simulink model "frbd_64ch_600mhz"  (R2013b)
settings: Solver=FixedStepDiscrete  SolverMode=SingleTasking  StartTime=0.0  StopTime=10.0  RelTol=1e-3
undefined symbols (not defined in the file): pfb_coeff_gen_calc
libraries: xbsIndex_r4 x14825, casper_library_delays x97, casper_library_misc x66, dspsigops x16, xps_library x5, casper_library_pfbs x2
(part 6 of 149)

== system frbd_64ch_600mhz/ACC6 ==
  addr : Inport
  data_in : Inport  Port=2
  we : Inport  Port=3
  calc_add : Subsystem  mask{data_width=32, addr_width=10, sample_rate=sample_rate}
      mask prompts: data_width "data width"; addr_width "address width"; sample_rate "sample rate"
  convert_addr : xbsIndex_r4/Convert  gui_display_data_type=Fixed-point  arith_type=Unsigned  n_bits=addr_width  bin_pt=0  float_type=Single  exp_bits=8  fraction_bits=24  quantization=Truncate  overflow=Wrap  en=off  latency=0  dbl_ovrd=off  pipeline=off  block_type=convert
      settings: xl_area=[0, 0, 0, 0, 0, 0, 0]
  convert_din1 : xbsIndex_r4/Convert  gui_display_data_type=Fixed-point  arith_type=Unsigned  n_bits=32  bin_pt=0  float_type=Single  exp_bits=8  fraction_bits=24  quantization=Truncate  overflow=Wrap  en=off  latency=0  dbl_ovrd=off  pipeline=off  block_type=convert
      settings: xl_area=[0, 0, 0, 0, 0, 0, 0]
  convert_we : xbsIndex_r4/Convert  gui_display_data_type=Fixed-point  arith_type=Unsigned  n_bits=1  bin_pt=0  float_type=Single  exp_bits=8  fraction_bits=24  quantization=Truncate  overflow=Wrap  en=off  latency=0  dbl_ovrd=off  pipeline=off  block_type=convert
      settings: xl_area=[0, 0, 0, 0, 0, 0, 0]
  frbd_64ch_600mhz_ACC6_addr : xbsIndex_r4/Gateway Out  inherit_from_input=off  hdl_port=on  timing_constraint=None  locs_specified=off  LOCs={'A5','B9','A9','C1','A3','G6','E9','A6','A7','A8','B8','B1','B3','D9','B5','B4','B6','C2'}  UseAsDAC=off  DACChannel='1'  block_type=gatewayout
      settings: infoedit="Gateway out block.  Converts Xilinx fixed point inputs into ouputs of type Simulink integer, double, or fixed point.<P><P>Hardware notes:  In hardware these blocks become top level output ports or are discarded, depending on how they are configured."  xl_area=[0, 0, 0, 0, 0, 0, 0]  sginterface={'Nallatech'=>{'xdspkit'=>{'non_memory_mapped_port'=>'uprev_Shared_BRAM_addr'}},'Xilinx'=>{'jtaghwcosim'=>{'non_memory_mapped_port'=>'uprev_Shared_BRAM_addr'},'xdspkit'=>{'non_memory_mapped_port'=>'uprev_Shared_BRAM_addr'}}}
  frbd_64ch_600mhz_ACC6_data_in : xbsIndex_r4/Gateway Out  inherit_from_input=off  hdl_port=on  timing_constraint=None  locs_specified=off  LOCs={'B21','B22','A22','B23','B19','C19','A20','A21','A23','B24','A24','A25','E18','D18','C18','B18'}  UseAsDAC=off  DACChannel='1'  block_type=gatewayout
      settings: infoedit="Gateway out block.  Converts Xilinx fixed point inputs into ouputs of type Simulink integer, double, or fixed point.<P><P>Hardware notes:  In hardware these blocks become top level output ports or are discarded, depending on how they are configured."  xl_area=[0, 0, 0, 0, 0, 0, 0]  sginterface={'Nallatech'=>{'xdspkit'=>{'non_memory_mapped_port'=>'uprev_Shared_BRAM_data_in'}},'Xilinx'=>{'jtaghwcosim'=>{'non_memory_mapped_port'=>'uprev_Shared_BRAM_data_in'},'xdspkit'=>{'non_memory_mapped_port'=>'uprev_Shared_BRAM_data_in'}}}
  frbd_64ch_600mhz_ACC6_data_out : xbsIndex_r4/Gateway In  gui_display_data_type=Fixed-point  arith_type=Unsigned  n_bits=32  bin_pt=0  preci_type=Single  exp_width=8  frac_width=24  quantization=Truncate  overflow=Wrap  period=sample_rate  dbl_ovrd=off  timing_constraint=None  locs_specified=off  LOCs={}  UseAsADC=off  ADCChannel='1'  inherit_from_input=off  hdl_port=on  block_type=gatewayin
      settings: xl_area=[0, 0, 0, 0, 0, 0, 0]
  frbd_64ch_600mhz_ACC6_we : xbsIndex_r4/Gateway Out  inherit_from_input=off  hdl_port=on  timing_constraint=None  locs_specified=off  LOCs={'A14'}  UseAsDAC=off  DACChannel='1'  block_type=gatewayout
      settings: infoedit="Gateway out block.  Converts Xilinx fixed point inputs into ouputs of type Simulink integer, double, or fixed point.<P><P>Hardware notes:  In hardware these blocks become top level output ports or are discarded, depending on how they are configured."  xl_area=[0, 0, 0, 0, 0, 0, 0]
  mem : Subsystem
  munge_in : Subsystem  AncestorBlock=casper_library_flow_control/munge  mask(munge){divisions=1, div_size=32, order=[0], arith_type_out=Unsigned, bin_pt_out=0}
      mask prompts: divisions "Number of divisions"; div_size "Division size (bits)"; order "Division packing order"; arith_type_out "Output arithmetic type"; bin_pt_out "Output binary point"
      mask help: Splits an input bus into the specified number of divisions and then recombines them in the order specified (most significant division = 0,least = number divisions-1)
      mask init:
      | munge_init(gcb, ...
      |     'divisions', divisions, ...
      |     'div_size', div_size, ...
      |     'order', order, ...
      |     'arith_type_out', arith_type_out, ...
      |     'bin_pt_out', bin_pt_out);
      settings: AttributesFormatString=|
      | split:32
      | join:0
      | Unsigned [32,0]
      mask TypeOptions arith_type_out: Unsigned | Signed  (2's comp) | Floating-point
  munge_out : Subsystem  AncestorBlock=casper_library_flow_control/munge  mask(munge){divisions=1, div_size=32, order=[0], arith_type_out=Unsigned, bin_pt_out=0}
      mask prompts: divisions "Number of divisions"; div_size "Division size (bits)"; order "Division packing order"; arith_type_out "Output arithmetic type"; bin_pt_out "Output binary point"
      mask help: Splits an input bus into the specified number of divisions and then recombines them in the order specified (most significant division = 0,least = number divisions-1)
      mask init:
      | munge_init(gcb, ...
      |     'divisions', divisions, ...
      |     'div_size', div_size, ...
      |     'order', order, ...
      |     'arith_type_out', arith_type_out, ...
      |     'bin_pt_out', bin_pt_out);
      settings: AttributesFormatString=|
      | split:32
      | join:0
      | Unsigned [32,0]
      mask TypeOptions arith_type_out: Unsigned | Signed  (2's comp) | Floating-point
  data_out : Outport
  wires:
  munge_in/1(dout) -> convert_din1/1
  munge_out/1(dout) -> data_out/1
  we/1 -> convert_we/1
  addr/1 -> calc_add/1(in)
  mem/1(Out1) -> frbd_64ch_600mhz_ACC6_data_out/1
  frbd_64ch_600mhz_ACC6_data_out/1 -> munge_out/1(din)
  convert_we/1 -> frbd_64ch_600mhz_ACC6_we/1
  frbd_64ch_600mhz_ACC6_addr/1 -> mem/1(In1)
  frbd_64ch_600mhz_ACC6_data_in/1 -> mem/2(In2)
  frbd_64ch_600mhz_ACC6_we/1 -> mem/3(In3)
  calc_add/1(out) -> convert_addr/1
  data_in/1 -> munge_in/1(din)
  convert_din1/1 -> frbd_64ch_600mhz_ACC6_data_in/1
  convert_addr/1 -> frbd_64ch_600mhz_ACC6_addr/1

== system frbd_64ch_600mhz/ACC7 ==
  addr : Inport
  data_in : Inport  Port=2
  we : Inport  Port=3
  calc_add : Subsystem  mask{data_width=32, addr_width=10, sample_rate=sample_rate}
      mask prompts: data_width "data width"; addr_width "address width"; sample_rate "sample rate"
  convert_addr : xbsIndex_r4/Convert  gui_display_data_type=Fixed-point  arith_type=Unsigned  n_bits=addr_width  bin_pt=0  float_type=Single  exp_bits=8  fraction_bits=24  quantization=Truncate  overflow=Wrap  en=off  latency=0  dbl_ovrd=off  pipeline=off  block_type=convert
      settings: xl_area=[0, 0, 0, 0, 0, 0, 0]
  convert_din1 : xbsIndex_r4/Convert  gui_display_data_type=Fixed-point  arith_type=Unsigned  n_bits=32  bin_pt=0  float_type=Single  exp_bits=8  fraction_bits=24  quantization=Truncate  overflow=Wrap  en=off  latency=0  dbl_ovrd=off  pipeline=off  block_type=convert
      settings: xl_area=[0, 0, 0, 0, 0, 0, 0]
  convert_we : xbsIndex_r4/Convert  gui_display_data_type=Fixed-point  arith_type=Unsigned  n_bits=1  bin_pt=0  float_type=Single  exp_bits=8  fraction_bits=24  quantization=Truncate  overflow=Wrap  en=off  latency=0  dbl_ovrd=off  pipeline=off  block_type=convert
      settings: xl_area=[0, 0, 0, 0, 0, 0, 0]
  frbd_64ch_600mhz_ACC7_addr : xbsIndex_r4/Gateway Out  inherit_from_input=off  hdl_port=on  timing_constraint=None  locs_specified=off  LOCs={'A5','B9','A9','C1','A3','G6','E9','A6','A7','A8','B8','B1','B3','D9','B5','B4','B6','C2'}  UseAsDAC=off  DACChannel='1'  block_type=gatewayout
      settings: infoedit="Gateway out block.  Converts Xilinx fixed point inputs into ouputs of type Simulink integer, double, or fixed point.<P><P>Hardware notes:  In hardware these blocks become top level output ports or are discarded, depending on how they are configured."  xl_area=[0, 0, 0, 0, 0, 0, 0]  sginterface={'Nallatech'=>{'xdspkit'=>{'non_memory_mapped_port'=>'uprev_Shared_BRAM_addr'}},'Xilinx'=>{'jtaghwcosim'=>{'non_memory_mapped_port'=>'uprev_Shared_BRAM_addr'},'xdspkit'=>{'non_memory_mapped_port'=>'uprev_Shared_BRAM_addr'}}}
  frbd_64ch_600mhz_ACC7_data_in : xbsIndex_r4/Gateway Out  inherit_from_input=off  hdl_port=on  timing_constraint=None  locs_specified=off  LOCs={'B21','B22','A22','B23','B19','C19','A20','A21','A23','B24','A24','A25','E18','D18','C18','B18'}  UseAsDAC=off  DACChannel='1'  block_type=gatewayout
      settings: infoedit="Gateway out block.  Converts Xilinx fixed point inputs into ouputs of type Simulink integer, double, or fixed point.<P><P>Hardware notes:  In hardware these blocks become top level output ports or are discarded, depending on how they are configured."  xl_area=[0, 0, 0, 0, 0, 0, 0]  sginterface={'Nallatech'=>{'xdspkit'=>{'non_memory_mapped_port'=>'uprev_Shared_BRAM_data_in'}},'Xilinx'=>{'jtaghwcosim'=>{'non_memory_mapped_port'=>'uprev_Shared_BRAM_data_in'},'xdspkit'=>{'non_memory_mapped_port'=>'uprev_Shared_BRAM_data_in'}}}
  frbd_64ch_600mhz_ACC7_data_out : xbsIndex_r4/Gateway In  gui_display_data_type=Fixed-point  arith_type=Unsigned  n_bits=32  bin_pt=0  preci_type=Single  exp_width=8  frac_width=24  quantization=Truncate  overflow=Wrap  period=sample_rate  dbl_ovrd=off  timing_constraint=None  locs_specified=off  LOCs={}  UseAsADC=off  ADCChannel='1'  inherit_from_input=off  hdl_port=on  block_type=gatewayin
      settings: xl_area=[0, 0, 0, 0, 0, 0, 0]
  frbd_64ch_600mhz_ACC7_we : xbsIndex_r4/Gateway Out  inherit_from_input=off  hdl_port=on  timing_constraint=None  locs_specified=off  LOCs={'A14'}  UseAsDAC=off  DACChannel='1'  block_type=gatewayout
      settings: infoedit="Gateway out block.  Converts Xilinx fixed point inputs into ouputs of type Simulink integer, double, or fixed point.<P><P>Hardware notes:  In hardware these blocks become top level output ports or are discarded, depending on how they are configured."  xl_area=[0, 0, 0, 0, 0, 0, 0]
  mem : Subsystem
  munge_in : Subsystem  AncestorBlock=casper_library_flow_control/munge  mask(munge){divisions=1, div_size=32, order=[0], arith_type_out=Unsigned, bin_pt_out=0}
      mask prompts: divisions "Number of divisions"; div_size "Division size (bits)"; order "Division packing order"; arith_type_out "Output arithmetic type"; bin_pt_out "Output binary point"
      mask help: Splits an input bus into the specified number of divisions and then recombines them in the order specified (most significant division = 0,least = number divisions-1)
      mask init:
      | munge_init(gcb, ...
      |     'divisions', divisions, ...
      |     'div_size', div_size, ...
      |     'order', order, ...
      |     'arith_type_out', arith_type_out, ...
      |     'bin_pt_out', bin_pt_out);
      settings: AttributesFormatString=|
      | split:32
      | join:0
      | Unsigned [32,0]
      mask TypeOptions arith_type_out: Unsigned | Signed  (2's comp) | Floating-point
  munge_out : Subsystem  AncestorBlock=casper_library_flow_control/munge  mask(munge){divisions=1, div_size=32, order=[0], arith_type_out=Unsigned, bin_pt_out=0}
      mask prompts: divisions "Number of divisions"; div_size "Division size (bits)"; order "Division packing order"; arith_type_out "Output arithmetic type"; bin_pt_out "Output binary point"
      mask help: Splits an input bus into the specified number of divisions and then recombines them in the order specified (most significant division = 0,least = number divisions-1)
      mask init:
      | munge_init(gcb, ...
      |     'divisions', divisions, ...
      |     'div_size', div_size, ...
      |     'order', order, ...
      |     'arith_type_out', arith_type_out, ...
      |     'bin_pt_out', bin_pt_out);
      settings: AttributesFormatString=|
      | split:32
      | join:0
      | Unsigned [32,0]
      mask TypeOptions arith_type_out: Unsigned | Signed  (2's comp) | Floating-point
  data_out : Outport
  wires:
  munge_in/1(dout) -> convert_din1/1
  munge_out/1(dout) -> data_out/1
  we/1 -> convert_we/1
  addr/1 -> calc_add/1(in)
  mem/1(Out1) -> frbd_64ch_600mhz_ACC7_data_out/1
  frbd_64ch_600mhz_ACC7_data_out/1 -> munge_out/1(din)
  convert_we/1 -> frbd_64ch_600mhz_ACC7_we/1
  frbd_64ch_600mhz_ACC7_addr/1 -> mem/1(In1)
  frbd_64ch_600mhz_ACC7_data_in/1 -> mem/2(In2)
  frbd_64ch_600mhz_ACC7_we/1 -> mem/3(In3)
  calc_add/1(out) -> convert_addr/1
  data_in/1 -> munge_in/1(din)
  convert_din1/1 -> frbd_64ch_600mhz_ACC7_data_in/1
  convert_addr/1 -> frbd_64ch_600mhz_ACC7_addr/1

== system frbd_64ch_600mhz/ACC8 ==
  addr : Inport
  data_in : Inport  Port=2
  we : Inport  Port=3
  calc_add : Subsystem  mask{data_width=32, addr_width=10, sample_rate=sample_rate}
      mask prompts: data_width "data width"; addr_width "address width"; sample_rate "sample rate"
  convert_addr : xbsIndex_r4/Convert  gui_display_data_type=Fixed-point  arith_type=Unsigned  n_bits=addr_width  bin_pt=0  float_type=Single  exp_bits=8  fraction_bits=24  quantization=Truncate  overflow=Wrap  en=off  latency=0  dbl_ovrd=off  pipeline=off  block_type=convert
      settings: xl_area=[0, 0, 0, 0, 0, 0, 0]
  convert_din1 : xbsIndex_r4/Convert  gui_display_data_type=Fixed-point  arith_type=Unsigned  n_bits=32  bin_pt=0  float_type=Single  exp_bits=8  fraction_bits=24  quantization=Truncate  overflow=Wrap  en=off  latency=0  dbl_ovrd=off  pipeline=off  block_type=convert
      settings: xl_area=[0, 0, 0, 0, 0, 0, 0]
  convert_we : xbsIndex_r4/Convert  gui_display_data_type=Fixed-point  arith_type=Unsigned  n_bits=1  bin_pt=0  float_type=Single  exp_bits=8  fraction_bits=24  quantization=Truncate  overflow=Wrap  en=off  latency=0  dbl_ovrd=off  pipeline=off  block_type=convert
      settings: xl_area=[0, 0, 0, 0, 0, 0, 0]
  frbd_64ch_600mhz_ACC8_addr : xbsIndex_r4/Gateway Out  inherit_from_input=off  hdl_port=on  timing_constraint=None  locs_specified=off  LOCs={'A5','B9','A9','C1','A3','G6','E9','A6','A7','A8','B8','B1','B3','D9','B5','B4','B6','C2'}  UseAsDAC=off  DACChannel='1'  block_type=gatewayout
      settings: infoedit="Gateway out block.  Converts Xilinx fixed point inputs into ouputs of type Simulink integer, double, or fixed point.<P><P>Hardware notes:  In hardware these blocks become top level output ports or are discarded, depending on how they are configured."  xl_area=[0, 0, 0, 0, 0, 0, 0]  sginterface={'Nallatech'=>{'xdspkit'=>{'non_memory_mapped_port'=>'uprev_Shared_BRAM_addr'}},'Xilinx'=>{'jtaghwcosim'=>{'non_memory_mapped_port'=>'uprev_Shared_BRAM_addr'},'xdspkit'=>{'non_memory_mapped_port'=>'uprev_Shared_BRAM_addr'}}}
  frbd_64ch_600mhz_ACC8_data_in : xbsIndex_r4/Gateway Out  inherit_from_input=off  hdl_port=on  timing_constraint=None  locs_specified=off  LOCs={'B21','B22','A22','B23','B19','C19','A20','A21','A23','B24','A24','A25','E18','D18','C18','B18'}  UseAsDAC=off  DACChannel='1'  block_type=gatewayout
      settings: infoedit="Gateway out block.  Converts Xilinx fixed point inputs into ouputs of type Simulink integer, double, or fixed point.<P><P>Hardware notes:  In hardware these blocks become top level output ports or are discarded, depending on how they are configured."  xl_area=[0, 0, 0, 0, 0, 0, 0]  sginterface={'Nallatech'=>{'xdspkit'=>{'non_memory_mapped_port'=>'uprev_Shared_BRAM_data_in'}},'Xilinx'=>{'jtaghwcosim'=>{'non_memory_mapped_port'=>'uprev_Shared_BRAM_data_in'},'xdspkit'=>{'non_memory_mapped_port'=>'uprev_Shared_BRAM_data_in'}}}
  frbd_64ch_600mhz_ACC8_data_out : xbsIndex_r4/Gateway In  gui_display_data_type=Fixed-point  arith_type=Unsigned  n_bits=32  bin_pt=0  preci_type=Single  exp_width=8  frac_width=24  quantization=Truncate  overflow=Wrap  period=sample_rate  dbl_ovrd=off  timing_constraint=None  locs_specified=off  LOCs={}  UseAsADC=off  ADCChannel='1'  inherit_from_input=off  hdl_port=on  block_type=gatewayin
      settings: xl_area=[0, 0, 0, 0, 0, 0, 0]
  frbd_64ch_600mhz_ACC8_we : xbsIndex_r4/Gateway Out  inherit_from_input=off  hdl_port=on  timing_constraint=None  locs_specified=off  LOCs={'A14'}  UseAsDAC=off  DACChannel='1'  block_type=gatewayout
      settings: infoedit="Gateway out block.  Converts Xilinx fixed point inputs into ouputs of type Simulink integer, double, or fixed point.<P><P>Hardware notes:  In hardware these blocks become top level output ports or are discarded, depending on how they are configured."  xl_area=[0, 0, 0, 0, 0, 0, 0]
  mem : Subsystem
  munge_in : Subsystem  AncestorBlock=casper_library_flow_control/munge  mask(munge){divisions=1, div_size=32, order=[0], arith_type_out=Unsigned, bin_pt_out=0}
      mask prompts: divisions "Number of divisions"; div_size "Division size (bits)"; order "Division packing order"; arith_type_out "Output arithmetic type"; bin_pt_out "Output binary point"
      mask help: Splits an input bus into the specified number of divisions and then recombines them in the order specified (most significant division = 0,least = number divisions-1)
      mask init:
      | munge_init(gcb, ...
      |     'divisions', divisions, ...
      |     'div_size', div_size, ...
      |     'order', order, ...
      |     'arith_type_out', arith_type_out, ...
      |     'bin_pt_out', bin_pt_out);
      settings: AttributesFormatString=|
      | split:32
      | join:0
      | Unsigned [32,0]
      mask TypeOptions arith_type_out: Unsigned | Signed  (2's comp) | Floating-point
  munge_out : Subsystem  AncestorBlock=casper_library_flow_control/munge  mask(munge){divisions=1, div_size=32, order=[0], arith_type_out=Unsigned, bin_pt_out=0}
      mask prompts: divisions "Number of divisions"; div_size "Division size (bits)"; order "Division packing order"; arith_type_out "Output arithmetic type"; bin_pt_out "Output binary point"
      mask help: Splits an input bus into the specified number of divisions and then recombines them in the order specified (most significant division = 0,least = number divisions-1)
      mask init:
      | munge_init(gcb, ...
      |     'divisions', divisions, ...
      |     'div_size', div_size, ...
      |     'order', order, ...
      |     'arith_type_out', arith_type_out, ...
      |     'bin_pt_out', bin_pt_out);
      settings: AttributesFormatString=|
      | split:32
      | join:0
      | Unsigned [32,0]
      mask TypeOptions arith_type_out: Unsigned | Signed  (2's comp) | Floating-point
  data_out : Outport
  wires:
  convert_addr/1 -> frbd_64ch_600mhz_ACC8_addr/1
  convert_din1/1 -> frbd_64ch_600mhz_ACC8_data_in/1
  data_in/1 -> munge_in/1(din)
  calc_add/1(out) -> convert_addr/1
  frbd_64ch_600mhz_ACC8_we/1 -> mem/3(In3)
  frbd_64ch_600mhz_ACC8_data_in/1 -> mem/2(In2)
  frbd_64ch_600mhz_ACC8_addr/1 -> mem/1(In1)
  convert_we/1 -> frbd_64ch_600mhz_ACC8_we/1
  frbd_64ch_600mhz_ACC8_data_out/1 -> munge_out/1(din)
  mem/1(Out1) -> frbd_64ch_600mhz_ACC8_data_out/1
  addr/1 -> calc_add/1(in)
  we/1 -> convert_we/1
  munge_out/1(dout) -> data_out/1
  munge_in/1(dout) -> convert_din1/1

== system frbd_64ch_600mhz/ACC9 ==
  addr : Inport
  data_in : Inport  Port=2
  we : Inport  Port=3
  calc_add : Subsystem  mask{data_width=32, addr_width=10, sample_rate=sample_rate}
      mask prompts: data_width "data width"; addr_width "address width"; sample_rate "sample rate"
  convert_addr : xbsIndex_r4/Convert  gui_display_data_type=Fixed-point  arith_type=Unsigned  n_bits=addr_width  bin_pt=0  float_type=Single  exp_bits=8  fraction_bits=24  quantization=Truncate  overflow=Wrap  en=off  latency=0  dbl_ovrd=off  pipeline=off  block_type=convert
      settings: xl_area=[0, 0, 0, 0, 0, 0, 0]
  convert_din1 : xbsIndex_r4/Convert  gui_display_data_type=Fixed-point  arith_type=Unsigned  n_bits=32  bin_pt=0  float_type=Single  exp_bits=8  fraction_bits=24  quantization=Truncate  overflow=Wrap  en=off  latency=0  dbl_ovrd=off  pipeline=off  block_type=convert
      settings: xl_area=[0, 0, 0, 0, 0, 0, 0]
  convert_we : xbsIndex_r4/Convert  gui_display_data_type=Fixed-point  arith_type=Unsigned  n_bits=1  bin_pt=0  float_type=Single  exp_bits=8  fraction_bits=24  quantization=Truncate  overflow=Wrap  en=off  latency=0  dbl_ovrd=off  pipeline=off  block_type=convert
      settings: xl_area=[0, 0, 0, 0, 0, 0, 0]
  frbd_64ch_600mhz_ACC9_addr : xbsIndex_r4/Gateway Out  inherit_from_input=off  hdl_port=on  timing_constraint=None  locs_specified=off  LOCs={'A5','B9','A9','C1','A3','G6','E9','A6','A7','A8','B8','B1','B3','D9','B5','B4','B6','C2'}  UseAsDAC=off  DACChannel='1'  block_type=gatewayout
      settings: infoedit="Gateway out block.  Converts Xilinx fixed point inputs into ouputs of type Simulink integer, double, or fixed point.<P><P>Hardware notes:  In hardware these blocks become top level output ports or are discarded, depending on how they are configured."  xl_area=[0, 0, 0, 0, 0, 0, 0]  sginterface={'Nallatech'=>{'xdspkit'=>{'non_memory_mapped_port'=>'uprev_Shared_BRAM_addr'}},'Xilinx'=>{'jtaghwcosim'=>{'non_memory_mapped_port'=>'uprev_Shared_BRAM_addr'},'xdspkit'=>{'non_memory_mapped_port'=>'uprev_Shared_BRAM_addr'}}}
  frbd_64ch_600mhz_ACC9_data_in : xbsIndex_r4/Gateway Out  inherit_from_input=off  hdl_port=on  timing_constraint=None  locs_specified=off  LOCs={'B21','B22','A22','B23','B19','C19','A20','A21','A23','B24','A24','A25','E18','D18','C18','B18'}  UseAsDAC=off  DACChannel='1'  block_type=gatewayout
      settings: infoedit="Gateway out block.  Converts Xilinx fixed point inputs into ouputs of type Simulink integer, double, or fixed point.<P><P>Hardware notes:  In hardware these blocks become top level output ports or are discarded, depending on how they are configured."  xl_area=[0, 0, 0, 0, 0, 0, 0]  sginterface={'Nallatech'=>{'xdspkit'=>{'non_memory_mapped_port'=>'uprev_Shared_BRAM_data_in'}},'Xilinx'=>{'jtaghwcosim'=>{'non_memory_mapped_port'=>'uprev_Shared_BRAM_data_in'},'xdspkit'=>{'non_memory_mapped_port'=>'uprev_Shared_BRAM_data_in'}}}
  frbd_64ch_600mhz_ACC9_data_out : xbsIndex_r4/Gateway In  gui_display_data_type=Fixed-point  arith_type=Unsigned  n_bits=32  bin_pt=0  preci_type=Single  exp_width=8  frac_width=24  quantization=Truncate  overflow=Wrap  period=sample_rate  dbl_ovrd=off  timing_constraint=None  locs_specified=off  LOCs={}  UseAsADC=off  ADCChannel='1'  inherit_from_input=off  hdl_port=on  block_type=gatewayin
      settings: xl_area=[0, 0, 0, 0, 0, 0, 0]
  frbd_64ch_600mhz_ACC9_we : xbsIndex_r4/Gateway Out  inherit_from_input=off  hdl_port=on  timing_constraint=None  locs_specified=off  LOCs={'A14'}  UseAsDAC=off  DACChannel='1'  block_type=gatewayout
      settings: infoedit="Gateway out block.  Converts Xilinx fixed point inputs into ouputs of type Simulink integer, double, or fixed point.<P><P>Hardware notes:  In hardware these blocks become top level output ports or are discarded, depending on how they are configured."  xl_area=[0, 0, 0, 0, 0, 0, 0]
  mem : Subsystem
  munge_in : Subsystem  AncestorBlock=casper_library_flow_control/munge  mask(munge){divisions=1, div_size=32, order=[0], arith_type_out=Unsigned, bin_pt_out=0}
      mask prompts: divisions "Number of divisions"; div_size "Division size (bits)"; order "Division packing order"; arith_type_out "Output arithmetic type"; bin_pt_out "Output binary point"
      mask help: Splits an input bus into the specified number of divisions and then recombines them in the order specified (most significant division = 0,least = number divisions-1)
      mask init:
      | munge_init(gcb, ...
      |     'divisions', divisions, ...
      |     'div_size', div_size, ...
      |     'order', order, ...
      |     'arith_type_out', arith_type_out, ...
      |     'bin_pt_out', bin_pt_out);
      settings: AttributesFormatString=|
      | split:32
      | join:0
      | Unsigned [32,0]
      mask TypeOptions arith_type_out: Unsigned | Signed  (2's comp) | Floating-point
  munge_out : Subsystem  AncestorBlock=casper_library_flow_control/munge  mask(munge){divisions=1, div_size=32, order=[0], arith_type_out=Unsigned, bin_pt_out=0}
      mask prompts: divisions "Number of divisions"; div_size "Division size (bits)"; order "Division packing order"; arith_type_out "Output arithmetic type"; bin_pt_out "Output binary point"
      mask help: Splits an input bus into the specified number of divisions and then recombines them in the order specified (most significant division = 0,least = number divisions-1)
      mask init:
      | munge_init(gcb, ...
      |     'divisions', divisions, ...
      |     'div_size', div_size, ...
      |     'order', order, ...
      |     'arith_type_out', arith_type_out, ...
      |     'bin_pt_out', bin_pt_out);
      settings: AttributesFormatString=|
      | split:32
      | join:0
      | Unsigned [32,0]
      mask TypeOptions arith_type_out: Unsigned | Signed  (2's comp) | Floating-point
  data_out : Outport
  wires:
  convert_addr/1 -> frbd_64ch_600mhz_ACC9_addr/1
  convert_din1/1 -> frbd_64ch_600mhz_ACC9_data_in/1
  data_in/1 -> munge_in/1(din)
  calc_add/1(out) -> convert_addr/1
  frbd_64ch_600mhz_ACC9_we/1 -> mem/3(In3)
  frbd_64ch_600mhz_ACC9_data_in/1 -> mem/2(In2)
  frbd_64ch_600mhz_ACC9_addr/1 -> mem/1(In1)
  convert_we/1 -> frbd_64ch_600mhz_ACC9_we/1
  frbd_64ch_600mhz_ACC9_data_out/1 -> munge_out/1(din)
  mem/1(Out1) -> frbd_64ch_600mhz_ACC9_data_out/1
  addr/1 -> calc_add/1(in)
  we/1 -> convert_we/1
  munge_out/1(dout) -> data_out/1
  munge_in/1(dout) -> convert_din1/1

== system frbd_64ch_600mhz/Parallel_Dedispersor_v1 ==
  Valid : Inport
  Data1 : Inport  Port=2
  Data2 : Inport  Port=3
  Data3 : Inport  Port=4
  Data4 : Inport  Port=5
  Dedispersor_v2_1 : Subsystem  mask(Detector de FRB (hasta 1024 canales)){DM_Vector=[0 11 22 33 43 52 60 68 75 82 88 94 99 104 109 113], behavioral=on}
      mask prompts: DM_Vector "DM Vector"; behavioral "behavioral delay"
      mask help:
      | Recibe un vector de DM asociado al retardo de cada canal y genera bloques detectores básicos para dedispersar la señal entregada.
      | Esta versión incorpora un contador de nbits en cada bloque de dedispersión.
      mask init:
      | config.source = str2func('honest_detector_v2');
      | config.toplevel = gcb;
      | config.depend = {'honest_detector_v2.m'};
      | xBlock(config, {DM_Vector, behavioral});
  Dedispersor_v2_2 : Subsystem  mask(Detector de FRB (hasta 1024 canales)){DM_Vector=[1 14 25 36 45 54 62 70 77 83 89 95 100 105 110 114], behavioral=on}
      mask prompts: DM_Vector "DM Vector"; behavioral "behavioral delay"
      mask help:
      | Recibe un vector de DM asociado al retardo de cada canal y genera bloques detectores básicos para dedispersar la señal entregada.
      | Esta versión incorpora un contador de nbits en cada bloque de dedispersión.
      mask init:
      | config.source = str2func('honest_detector_v2');
      | config.toplevel = gcb;
      | config.depend = {'honest_detector_v2.m'};
      | xBlock(config, {DM_Vector, behavioral});
  Dedispersor_v2_3 : Subsystem  mask(Detector de FRB (hasta 1024 canales)){DM_Vector=[4 17 28 38 47 56 64 72 78 85 91 96 101 106 111 115], behavioral=on}
      mask prompts: DM_Vector "DM Vector"; behavioral "behavioral delay"
      mask help:
      | Recibe un vector de DM asociado al retardo de cada canal y genera bloques detectores básicos para dedispersar la señal entregada.
      | Esta versión incorpora un contador de nbits en cada bloque de dedispersión.
      mask init:
      | config.source = str2func('honest_detector_v2');
      | config.toplevel = gcb;
      | config.depend = {'honest_detector_v2.m'};
      | xBlock(config, {DM_Vector, behavioral});
  Dedispersor_v2_4 : Subsystem  mask(Detector de FRB (hasta 1024 canales)){DM_Vector=[7 19 30 40 50 58 66 73 80 86 92 98 103 107 112 116], behavioral=on}
      mask prompts: DM_Vector "DM Vector"; behavioral "behavioral delay"
      mask help:
      | Recibe un vector de DM asociado al retardo de cada canal y genera bloques detectores básicos para dedispersar la señal entregada.
      | Esta versión incorpora un contador de nbits en cada bloque de dedispersión.
      mask init:
      | config.source = str2func('honest_detector_v2');
      | config.toplevel = gcb;
      | config.depend = {'honest_detector_v2.m'};
      | xBlock(config, {DM_Vector, behavioral});
  Out1 : Outport
  Out2 : Outport  Port=2
  Out3 : Outport  Port=3
  Out4 : Outport  Port=4
  wires:
  Valid/1 -> Dedispersor_v2_1/2(Valid), Dedispersor_v2_2/2(Valid), Dedispersor_v2_3/2(Valid), Dedispersor_v2_4/2(Valid)
  Data1/1 -> Dedispersor_v2_1/1(Data)
  Data2/1 -> Dedispersor_v2_2/1(Data)
  Data3/1 -> Dedispersor_v2_3/1(Data)
  Data4/1 -> Dedispersor_v2_4/1(Data)
  Dedispersor_v2_1/1(Output) -> Out1/1
  Dedispersor_v2_2/1(Output) -> Out2/1
  Dedispersor_v2_3/1(Output) -> Out3/1
  Dedispersor_v2_4/1(Output) -> Out4/1

== system frbd_64ch_600mhz/Parallel_Dedispersor_v11 ==
  Valid : Inport
  Data1 : Inport  Port=2
  Data2 : Inport  Port=3
  Data3 : Inport  Port=4
  Data4 : Inport  Port=5
  Dedispersor_v2_1 : Subsystem  mask(Detector de FRB (hasta 1024 canales)){DM_Vector=[0 11 22 33 43 52 60 68 75 82 88 94 99 104 109 113], behavioral=on}
      mask prompts: DM_Vector "DM Vector"; behavioral "behavioral delay"
      mask help:
      | Recibe un vector de DM asociado al retardo de cada canal y genera bloques detectores básicos para dedispersar la señal entregada.
      | Esta versión incorpora un contador de nbits en cada bloque de dedispersión.
      mask init:
      | config.source = str2func('honest_detector_v2');
      | config.toplevel = gcb;
      | config.depend = {'honest_detector_v2.m'};
      | xBlock(config, {DM_Vector, behavioral});
  Dedispersor_v2_2 : Subsystem  mask(Detector de FRB (hasta 1024 canales)){DM_Vector=[1 14 25 36 45 54 62 70 77 83 89 95 100 105 110 114], behavioral=on}
      mask prompts: DM_Vector "DM Vector"; behavioral "behavioral delay"
      mask help:
      | Recibe un vector de DM asociado al retardo de cada canal y genera bloques detectores básicos para dedispersar la señal entregada.
      | Esta versión incorpora un contador de nbits en cada bloque de dedispersión.
      mask init:
      | config.source = str2func('honest_detector_v2');
      | config.toplevel = gcb;
      | config.depend = {'honest_detector_v2.m'};
      | xBlock(config, {DM_Vector, behavioral});
  Dedispersor_v2_3 : Subsystem  mask(Detector de FRB (hasta 1024 canales)){DM_Vector=[4 17 28 38 47 56 64 72 78 85 91 96 101 106 111 115], behavioral=on}
      mask prompts: DM_Vector "DM Vector"; behavioral "behavioral delay"
      mask help:
      | Recibe un vector de DM asociado al retardo de cada canal y genera bloques detectores básicos para dedispersar la señal entregada.
      | Esta versión incorpora un contador de nbits en cada bloque de dedispersión.
      mask init:
      | config.source = str2func('honest_detector_v2');
      | config.toplevel = gcb;
      | config.depend = {'honest_detector_v2.m'};
      | xBlock(config, {DM_Vector, behavioral});
  Dedispersor_v2_4 : Subsystem  mask(Detector de FRB (hasta 1024 canales)){DM_Vector=[7 19 30 40 50 58 66 73 80 86 92 98 103 107 112 116], behavioral=on}
      mask prompts: DM_Vector "DM Vector"; behavioral "behavioral delay"
      mask help:
      | Recibe un vector de DM asociado al retardo de cada canal y genera bloques detectores básicos para dedispersar la señal entregada.
      | Esta versión incorpora un contador de nbits en cada bloque de dedispersión.
      mask init:
      | config.source = str2func('honest_detector_v2');
      | config.toplevel = gcb;
      | config.depend = {'honest_detector_v2.m'};
      | xBlock(config, {DM_Vector, behavioral});
  Out1 : Outport
  Out2 : Outport  Port=2
  Out3 : Outport  Port=3
  Out4 : Outport  Port=4
  wires:
  Valid/1 -> Dedispersor_v2_3/2(Valid), Dedispersor_v2_4/2(Valid), Dedispersor_v2_2/2(Valid), Dedispersor_v2_1/2(Valid)
  Data1/1 -> Dedispersor_v2_1/1(Data)
  Data2/1 -> Dedispersor_v2_2/1(Data)
  Data3/1 -> Dedispersor_v2_3/1(Data)
  Data4/1 -> Dedispersor_v2_4/1(Data)
  Dedispersor_v2_1/1(Output) -> Out1/1
  Dedispersor_v2_2/1(Output) -> Out2/1
  Dedispersor_v2_3/1(Output) -> Out3/1
  Dedispersor_v2_4/1(Output) -> Out4/1

== system frbd_64ch_600mhz/Parallel_Dedispersor_v2 ==
  Valid : Inport
  Data1 : Inport  Port=2
  Data2 : Inport  Port=3
  Data3 : Inport  Port=4
  Data4 : Inport  Port=5
  Dedispersor_v2_1 : Subsystem  mask(Detector de FRB (hasta 1024 canales)){DM_Vector=[0 11 22 33 43 52 60 68 75 82 88 94 99 104 109 113], behavioral=on}
      mask prompts: DM_Vector "DM Vector"; behavioral "behavioral delay"
      mask help:
      | Recibe un vector de DM asociado al retardo de cada canal y genera bloques detectores básicos para dedispersar la señal entregada.
      | Esta versión incorpora un contador de nbits en cada bloque de dedispersión.
      mask init:
      | config.source = str2func('honest_detector_v2');
      | config.toplevel = gcb;
      | config.depend = {'honest_detector_v2.m'};
      | xBlock(config, {DM_Vector, behavioral});
  Dedispersor_v2_2 : Subsystem  mask(Detector de FRB (hasta 1024 canales)){DM_Vector=[1 14 25 36 45 54 62 70 77 83 89 95 100 105 110 114], behavioral=on}
      mask prompts: DM_Vector "DM Vector"; behavioral "behavioral delay"
      mask help:
      | Recibe un vector de DM asociado al retardo de cada canal y genera bloques detectores básicos para dedispersar la señal entregada.
      | Esta versión incorpora un contador de nbits en cada bloque de dedispersión.
      mask init:
      | config.source = str2func('honest_detector_v2');
      | config.toplevel = gcb;
      | config.depend = {'honest_detector_v2.m'};
      | xBlock(config, {DM_Vector, behavioral});
  Dedispersor_v2_3 : Subsystem  mask(Detector de FRB (hasta 1024 canales)){DM_Vector=[4 17 28 38 47 56 64 72 78 85 91 96 101 106 111 115], behavioral=on}
      mask prompts: DM_Vector "DM Vector"; behavioral "behavioral delay"
      mask help:
      | Recibe un vector de DM asociado al retardo de cada canal y genera bloques detectores básicos para dedispersar la señal entregada.
      | Esta versión incorpora un contador de nbits en cada bloque de dedispersión.
      mask init:
      | config.source = str2func('honest_detector_v2');
      | config.toplevel = gcb;
      | config.depend = {'honest_detector_v2.m'};
      | xBlock(config, {DM_Vector, behavioral});
  Dedispersor_v2_4 : Subsystem  mask(Detector de FRB (hasta 1024 canales)){DM_Vector=[7 19 30 40 50 58 66 73 80 86 92 98 103 107 112 116], behavioral=on}
      mask prompts: DM_Vector "DM Vector"; behavioral "behavioral delay"
      mask help:
      | Recibe un vector de DM asociado al retardo de cada canal y genera bloques detectores básicos para dedispersar la señal entregada.
      | Esta versión incorpora un contador de nbits en cada bloque de dedispersión.
      mask init:
      | config.source = str2func('honest_detector_v2');
      | config.toplevel = gcb;
      | config.depend = {'honest_detector_v2.m'};
      | xBlock(config, {DM_Vector, behavioral});
  Out1 : Outport
  Out2 : Outport  Port=2
  Out3 : Outport  Port=3
  Out4 : Outport  Port=4
  wires:
  Valid/1 -> Dedispersor_v2_1/2(Valid), Dedispersor_v2_2/2(Valid), Dedispersor_v2_3/2(Valid), Dedispersor_v2_4/2(Valid)
  Data1/1 -> Dedispersor_v2_1/1(Data)
  Data2/1 -> Dedispersor_v2_2/1(Data)
  Data3/1 -> Dedispersor_v2_3/1(Data)
  Data4/1 -> Dedispersor_v2_4/1(Data)
  Dedispersor_v2_1/1(Output) -> Out1/1
  Dedispersor_v2_2/1(Output) -> Out2/1
  Dedispersor_v2_3/1(Output) -> Out3/1
  Dedispersor_v2_4/1(Output) -> Out4/1

== system frbd_64ch_600mhz/Parallel_Dedispersor_v3 ==
  Valid : Inport
  Data1 : Inport  Port=2
  Data2 : Inport  Port=3
  Data3 : Inport  Port=4
  Data4 : Inport  Port=5
  Dedispersor_v2_1 : Subsystem  mask(Detector de FRB (hasta 1024 canales)){DM_Vector=[0 11 22 33 43 52 60 68 75 82 88 94 99 104 109 113], behavioral=on}
      mask prompts: DM_Vector "DM Vector"; behavioral "behavioral delay"
      mask help:
      | Recibe un vector de DM asociado al retardo de cada canal y genera bloques detectores básicos para dedispersar la señal entregada.
      | Esta versión incorpora un contador de nbits en cada bloque de dedispersión.
      mask init:
      | config.source = str2func('honest_detector_v2');
      | config.toplevel = gcb;
      | config.depend = {'honest_detector_v2.m'};
      | xBlock(config, {DM_Vector, behavioral});
  Dedispersor_v2_2 : Subsystem  mask(Detector de FRB (hasta 1024 canales)){DM_Vector=[1 14 25 36 45 54 62 70 77 83 89 95 100 105 110 114], behavioral=on}
      mask prompts: DM_Vector "DM Vector"; behavioral "behavioral delay"
      mask help:
      | Recibe un vector de DM asociado al retardo de cada canal y genera bloques detectores básicos para dedispersar la señal entregada.
      | Esta versión incorpora un contador de nbits en cada bloque de dedispersión.
      mask init:
      | config.source = str2func('honest_detector_v2');
      | config.toplevel = gcb;
      | config.depend = {'honest_detector_v2.m'};
      | xBlock(config, {DM_Vector, behavioral});
  Dedispersor_v2_3 : Subsystem  mask(Detector de FRB (hasta 1024 canales)){DM_Vector=[4 17 28 38 47 56 64 72 78 85 91 96 101 106 111 115], behavioral=on}
      mask prompts: DM_Vector "DM Vector"; behavioral "behavioral delay"
      mask help:
      | Recibe un vector de DM asociado al retardo de cada canal y genera bloques detectores básicos para dedispersar la señal entregada.
      | Esta versión incorpora un contador de nbits en cada bloque de dedispersión.
      mask init:
      | config.source = str2func('honest_detector_v2');
      | config.toplevel = gcb;
      | config.depend = {'honest_detector_v2.m'};
      | xBlock(config, {DM_Vector, behavioral});
  Dedispersor_v2_4 : Subsystem  mask(Detector de FRB (hasta 1024 canales)){DM_Vector=[7 19 30 40 50 58 66 73 80 86 92 98 103 107 112 116], behavioral=on}
      mask prompts: DM_Vector "DM Vector"; behavioral "behavioral delay"
      mask help:
      | Recibe un vector de DM asociado al retardo de cada canal y genera bloques detectores básicos para dedispersar la señal entregada.
      | Esta versión incorpora un contador de nbits en cada bloque de dedispersión.
      mask init:
      | config.source = str2func('honest_detector_v2');
      | config.toplevel = gcb;
      | config.depend = {'honest_detector_v2.m'};
      | xBlock(config, {DM_Vector, behavioral});
  Out1 : Outport
  Out2 : Outport  Port=2
  Out3 : Outport  Port=3
  Out4 : Outport  Port=4
  wires:
  Valid/1 -> Dedispersor_v2_1/2(Valid), Dedispersor_v2_2/2(Valid), Dedispersor_v2_3/2(Valid), Dedispersor_v2_4/2(Valid)
  Data1/1 -> Dedispersor_v2_1/1(Data)
  Data2/1 -> Dedispersor_v2_2/1(Data)
  Data3/1 -> Dedispersor_v2_3/1(Data)
  Data4/1 -> Dedispersor_v2_4/1(Data)
  Dedispersor_v2_1/1(Output) -> Out1/1
  Dedispersor_v2_2/1(Output) -> Out2/1
  Dedispersor_v2_3/1(Output) -> Out3/1
  Dedispersor_v2_4/1(Output) -> Out4/1

== system frbd_64ch_600mhz/Parallel_Dedispersor_v4 ==
  Valid : Inport
  Data1 : Inport  Port=2
  Data2 : Inport  Port=3
  Data3 : Inport  Port=4
  Data4 : Inport  Port=5
  Dedispersor_v2_1 : Subsystem  mask(Detector de FRB (hasta 1024 canales)){DM_Vector=[0 11 22 33 43 52 60 68 75 82 88 94 99 104 109 113], behavioral=on}
      mask prompts: DM_Vector "DM Vector"; behavioral "behavioral delay"
      mask help:
      | Recibe un vector de DM asociado al retardo de cada canal y genera bloques detectores básicos para dedispersar la señal entregada.
      | Esta versión incorpora un contador de nbits en cada bloque de dedispersión.
      mask init:
      | config.source = str2func('honest_detector_v2');
      | config.toplevel = gcb;
      | config.depend = {'honest_detector_v2.m'};
      | xBlock(config, {DM_Vector, behavioral});
  Dedispersor_v2_2 : Subsystem  mask(Detector de FRB (hasta 1024 canales)){DM_Vector=[1 14 25 36 45 54 62 70 77 83 89 95 100 105 110 114], behavioral=on}
      mask prompts: DM_Vector "DM Vector"; behavioral "behavioral delay"
      mask help:
      | Recibe un vector de DM asociado al retardo de cada canal y genera bloques detectores básicos para dedispersar la señal entregada.
      | Esta versión incorpora un contador de nbits en cada bloque de dedispersión.
      mask init:
      | config.source = str2func('honest_detector_v2');
      | config.toplevel = gcb;
      | config.depend = {'honest_detector_v2.m'};
      | xBlock(config, {DM_Vector, behavioral});
  Dedispersor_v2_3 : Subsystem  mask(Detector de FRB (hasta 1024 canales)){DM_Vector=[4 17 28 38 47 56 64 72 78 85 91 96 101 106 111 115], behavioral=on}
      mask prompts: DM_Vector "DM Vector"; behavioral "behavioral delay"
      mask help:
      | Recibe un vector de DM asociado al retardo de cada canal y genera bloques detectores básicos para dedispersar la señal entregada.
      | Esta versión incorpora un contador de nbits en cada bloque de dedispersión.
      mask init:
      | config.source = str2func('honest_detector_v2');
      | config.toplevel = gcb;
      | config.depend = {'honest_detector_v2.m'};
      | xBlock(config, {DM_Vector, behavioral});
  Dedispersor_v2_4 : Subsystem  mask(Detector de FRB (hasta 1024 canales)){DM_Vector=[7 19 30 40 50 58 66 73 80 86 92 98 103 107 112 116], behavioral=on}
      mask prompts: DM_Vector "DM Vector"; behavioral "behavioral delay"
      mask help:
      | Recibe un vector de DM asociado al retardo de cada canal y genera bloques detectores básicos para dedispersar la señal entregada.
      | Esta versión incorpora un contador de nbits en cada bloque de dedispersión.
      mask init:
      | config.source = str2func('honest_detector_v2');
      | config.toplevel = gcb;
      | config.depend = {'honest_detector_v2.m'};
      | xBlock(config, {DM_Vector, behavioral});
  Out1 : Outport
  Out2 : Outport  Port=2
  Out3 : Outport  Port=3
  Out4 : Outport  Port=4
  wires:
  Valid/1 -> Dedispersor_v2_1/2(Valid), Dedispersor_v2_2/2(Valid), Dedispersor_v2_3/2(Valid), Dedispersor_v2_4/2(Valid)
  Data1/1 -> Dedispersor_v2_1/1(Data)
  Data2/1 -> Dedispersor_v2_2/1(Data)
  Data3/1 -> Dedispersor_v2_3/1(Data)
  Data4/1 -> Dedispersor_v2_4/1(Data)
  Dedispersor_v2_1/1(Output) -> Out1/1
  Dedispersor_v2_2/1(Output) -> Out2/1
  Dedispersor_v2_3/1(Output) -> Out3/1
  Dedispersor_v2_4/1(Output) -> Out4/1

== system frbd_64ch_600mhz/Parallel_Dedispersor_v5 ==
  Valid : Inport
  Data1 : Inport  Port=2
  Data2 : Inport  Port=3
  Data3 : Inport  Port=4
  Data4 : Inport  Port=5
  Dedispersor_v2_1 : Subsystem  mask(Detector de FRB (hasta 1024 canales)){DM_Vector=[0 11 22 33 43 52 60 68 75 82 88 94 99 104 109 113], behavioral=on}
      mask prompts: DM_Vector "DM Vector"; behavioral "behavioral delay"
      mask help:
      | Recibe un vector de DM asociado al retardo de cada canal y genera bloques detectores básicos para dedispersar la señal entregada.
      | Esta versión incorpora un contador de nbits en cada bloque de dedispersión.
      mask init:
      | config.source = str2func('honest_detector_v2');
      | config.toplevel = gcb;
      | config.depend = {'honest_detector_v2.m'};
      | xBlock(config, {DM_Vector, behavioral});
  Dedispersor_v2_2 : Subsystem  mask(Detector de FRB (hasta 1024 canales)){DM_Vector=[1 14 25 36 45 54 62 70 77 83 89 95 100 105 110 114], behavioral=on}
      mask prompts: DM_Vector "DM Vector"; behavioral "behavioral delay"
      mask help:
      | Recibe un vector de DM asociado al retardo de cada canal y genera bloques detectores básicos para dedispersar la señal entregada.
      | Esta versión incorpora un contador de nbits en cada bloque de dedispersión.
      mask init:
      | config.source = str2func('honest_detector_v2');
      | config.toplevel = gcb;
      | config.depend = {'honest_detector_v2.m'};
      | xBlock(config, {DM_Vector, behavioral});
  Dedispersor_v2_3 : Subsystem  mask(Detector de FRB (hasta 1024 canales)){DM_Vector=[4 17 28 38 47 56 64 72 78 85 91 96 101 106 111 115], behavioral=on}
      mask prompts: DM_Vector "DM Vector"; behavioral "behavioral delay"
      mask help:
      | Recibe un vector de DM asociado al retardo de cada canal y genera bloques detectores básicos para dedispersar la señal entregada.
      | Esta versión incorpora un contador de nbits en cada bloque de dedispersión.
      mask init:
      | config.source = str2func('honest_detector_v2');
      | config.toplevel = gcb;
      | config.depend = {'honest_detector_v2.m'};
      | xBlock(config, {DM_Vector, behavioral});
  Dedispersor_v2_4 : Subsystem  mask(Detector de FRB (hasta 1024 canales)){DM_Vector=[7 19 30 40 50 58 66 73 80 86 92 98 103 107 112 116], behavioral=on}
      mask prompts: DM_Vector "DM Vector"; behavioral "behavioral delay"
      mask help:
      | Recibe un vector de DM asociado al retardo de cada canal y genera bloques detectores básicos para dedispersar la señal entregada.
      | Esta versión incorpora un contador de nbits en cada bloque de dedispersión.
      mask init:
      | config.source = str2func('honest_detector_v2');
      | config.toplevel = gcb;
      | config.depend = {'honest_detector_v2.m'};
      | xBlock(config, {DM_Vector, behavioral});
  Out1 : Outport
  Out2 : Outport  Port=2
  Out3 : Outport  Port=3
  Out4 : Outport  Port=4
  wires:
  Valid/1 -> Dedispersor_v2_1/2(Valid), Dedispersor_v2_2/2(Valid), Dedispersor_v2_3/2(Valid), Dedispersor_v2_4/2(Valid)
  Data1/1 -> Dedispersor_v2_1/1(Data)
  Data2/1 -> Dedispersor_v2_2/1(Data)
  Data3/1 -> Dedispersor_v2_3/1(Data)
  Data4/1 -> Dedispersor_v2_4/1(Data)
  Dedispersor_v2_1/1(Output) -> Out1/1
  Dedispersor_v2_2/1(Output) -> Out2/1
  Dedispersor_v2_3/1(Output) -> Out3/1
  Dedispersor_v2_4/1(Output) -> Out4/1

== system frbd_64ch_600mhz/Parallel_Dedispersor_v6 ==
  Valid : Inport
  Data1 : Inport  Port=2
  Data2 : Inport  Port=3
  Data3 : Inport  Port=4
  Data4 : Inport  Port=5
  Dedispersor_v2_1 : Subsystem  mask(Detector de FRB (hasta 1024 canales)){DM_Vector=[0 11 22 33 43 52 60 68 75 82 88 94 99 104 109 113], behavioral=on}
      mask prompts: DM_Vector "DM Vector"; behavioral "behavioral delay"
      mask help:
      | Recibe un vector de DM asociado al retardo de cada canal y genera bloques detectores básicos para dedispersar la señal entregada.
      | Esta versión incorpora un contador de nbits en cada bloque de dedispersión.
      mask init:
      | config.source = str2func('honest_detector_v2');
      | config.toplevel = gcb;
      | config.depend = {'honest_detector_v2.m'};
      | xBlock(config, {DM_Vector, behavioral});
  Dedispersor_v2_2 : Subsystem  mask(Detector de FRB (hasta 1024 canales)){DM_Vector=[1 14 25 36 45 54 62 70 77 83 89 95 100 105 110 114], behavioral=on}
      mask prompts: DM_Vector "DM Vector"; behavioral "behavioral delay"
      mask help:
      | Recibe un vector de DM asociado al retardo de cada canal y genera bloques detectores básicos para dedispersar la señal entregada.
      | Esta versión incorpora un contador de nbits en cada bloque de dedispersión.
      mask init:
      | config.source = str2func('honest_detector_v2');
      | config.toplevel = gcb;
      | config.depend = {'honest_detector_v2.m'};
      | xBlock(config, {DM_Vector, behavioral});
  Dedispersor_v2_3 : Subsystem  mask(Detector de FRB (hasta 1024 canales)){DM_Vector=[4 17 28 38 47 56 64 72 78 85 91 96 101 106 111 115], behavioral=on}
      mask prompts: DM_Vector "DM Vector"; behavioral "behavioral delay"
      mask help:
      | Recibe un vector de DM asociado al retardo de cada canal y genera bloques detectores básicos para dedispersar la señal entregada.
      | Esta versión incorpora un contador de nbits en cada bloque de dedispersión.
      mask init:
      | config.source = str2func('honest_detector_v2');
      | config.toplevel = gcb;
      | config.depend = {'honest_detector_v2.m'};
      | xBlock(config, {DM_Vector, behavioral});
  Dedispersor_v2_4 : Subsystem  mask(Detector de FRB (hasta 1024 canales)){DM_Vector=[7 19 30 40 50 58 66 73 80 86 92 98 103 107 112 116], behavioral=on}
      mask prompts: DM_Vector "DM Vector"; behavioral "behavioral delay"
      mask help:
      | Recibe un vector de DM asociado al retardo de cada canal y genera bloques detectores básicos para dedispersar la señal entregada.
      | Esta versión incorpora un contador de nbits en cada bloque de dedispersión.
      mask init:
      | config.source = str2func('honest_detector_v2');
      | config.toplevel = gcb;
      | config.depend = {'honest_detector_v2.m'};
      | xBlock(config, {DM_Vector, behavioral});
  Out1 : Outport
  Out2 : Outport  Port=2
  Out3 : Outport  Port=3
  Out4 : Outport  Port=4
  wires:
  Valid/1 -> Dedispersor_v2_1/2(Valid), Dedispersor_v2_2/2(Valid), Dedispersor_v2_3/2(Valid), Dedispersor_v2_4/2(Valid)
  Data1/1 -> Dedispersor_v2_1/1(Data)
  Data2/1 -> Dedispersor_v2_2/1(Data)
  Data3/1 -> Dedispersor_v2_3/1(Data)
  Data4/1 -> Dedispersor_v2_4/1(Data)
  Dedispersor_v2_1/1(Output) -> Out1/1
  Dedispersor_v2_2/1(Output) -> Out2/1
  Dedispersor_v2_3/1(Output) -> Out3/1
  Dedispersor_v2_4/1(Output) -> Out4/1
